simulink model "INPUT_autosar"  (R2019b)
settings: Solver=FixedStepAuto  StartTime=0.0  StopTime=10.0  RelTol=1e-3
undefined symbols (not defined in the file or in its folder): I_AN07_5V, I_AN08_5V, I_AN10_5V, I_SW01_L, I_SW02_L, I_SW03_L
libraries: ec5744lib x51, canmsglib x13
(part 1 of 2)
settings Model: Creator=12045  LastModifiedBy=12045
settings DataIOCC: ReturnWorkspaceOutputs=off
settings OptimizationCC: DefaultParameterBehavior=Inlined  EnhancedBackFolding=on  PassReuseOutputArgsAs=Individual arguments  ZeroExternalMemoryAtStartup=off  ZeroInternalMemoryAtStartup=off  OptimizeBlockOrder=speed  DifferentSizesBufferReuse=on  OptimizationCustomize=off  EfficientTunableParamExpr=on
settings DebuggingCC: ParameterTunabilityLossMsg=error  ArithmeticOperatorsInVariantConditions=warning
settings SFSimCC: MATLABDynamicMemAlloc=off  CustomCodeUndefinedFunction=UseInterfaceOnly
settings RTWCC: Description=AUTOSAR  SystemTargetFile=autosar.tlc  GenCodeOnly=on  TemplateMakefile=ert_default_tmf  GenerateReport=on  IncludeHyperlinkInReport=on  LaunchReport=on  GenerateTraceInfo=on  GenerateTraceReport=on  GenerateTraceReportSl=on  GenerateTraceReportSf=on  GenerateTraceReportEml=on
settings CodeAppCC: ForceParamTrailComments=on  IgnoreCustomStorageClasses=off  OperatorAnnotations=on  SimulinkDataObjDesc=on  SFDataObjDesc=on  InsertBlockDesc=on
settings STFCustomTargetCC: TargetLangStandard=C99 (ISO)  MultiwordLength=256  ParMdlRefBuildCompliant=on  CompOptLevelCompliant=on  IncludeMdlTerminateFcn=off  CombineOutputUpdateFcns=on  SuppressErrorStatus=on  ERTCustomFileBanners=on  SupportNonFinite=off  SupportComplex=off  SupportContinuousTime=off  SupportNonInlinedSFcns=off  RemoveResetFunc=on  MATLABClassNameForMDSCustomization=Simulink.SoftwareTarget.ERTCustomization  AutosarCompliant=on  UseToolchainInfoCompliant=on  LookupTableObjectStructAxisOrder=2,1,3,4,...  LUTObjectStructOrderEvenSpacing=Size,Table,Breakpoints  SystemTargetFile=autosar.tlc
settings ERTTargetCC: TargetLangStandard=C99 (ISO)  ConcurrentExecutionCompliant=off  IncludeMdlTerminateFcn=off  SuppressErrorStatus=on  SupportNonFinite=off  SupportComplex=off  ModelStepFunctionPrototypeControlCompliant=off  CPPClassGenCompliant=off  AutosarCompliant=on  LookupTableObjectStructAxisOrder=2,1,3,4,...  LUTObjectStructOrderEvenSpacing=Size,Table,Breakpoints  InlinedParameterPlacement=NonHierarchical  ERTCustomFileTemplate=example_file_process.tlc

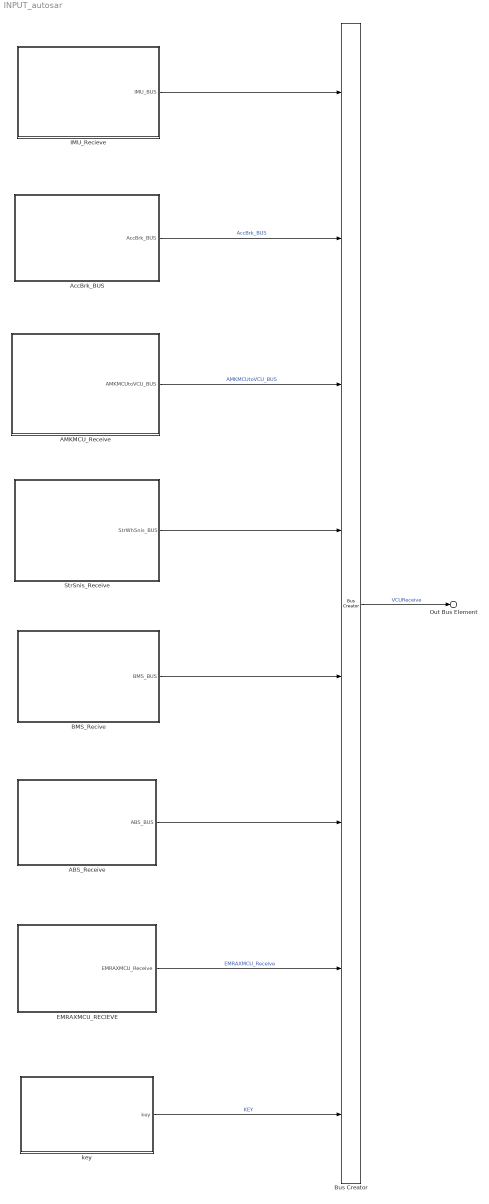
== system INPUT_autosar ==
  ABS_Receive : Subsystem  TreatAsAtomicUnit=on
  AMKMCU_Receive : Subsystem
  AccBrk_BUS : Subsystem
  BMS_Recive : Subsystem  TreatAsAtomicUnit=on
  Bus Creator : BusCreator  Inputs=8
  EMRAXMCU_RECIEVE : Subsystem  TreatAsAtomicUnit=on
  IMU_Recieve : Subsystem  TreatAsAtomicUnit=on
  StrSnis_Receive : Subsystem  TreatAsAtomicUnit=on
  key : Subsystem  TreatAsAtomicUnit=on
  Out Bus Element : Outport  PortName=INPUT_BUS  Element=INPUT_BUS
  wires:
  ABS_Receive/1(ABS_BUS) -> Bus Creator/6
  key/1(key) -> Bus Creator/8  "KEY"
  AMKMCU_Receive/1(AMKMCUtoVCU_BUS) -> Bus Creator/3  "AMKMCUtoVCU_BUS"
  BMS_Recive/1(BMS_BUS) -> Bus Creator/5
  AccBrk_BUS/1(AccBrk_BUS) -> Bus Creator/2  "AccBrk_BUS"
  IMU_Recieve/1(IMU_BUS) -> Bus Creator/1
  EMRAXMCU_RECIEVE/1(EMRAXMCU_Receive) -> Bus Creator/7  "EMRAXMCU_Receive"
  StrSnis_Receive/1(StrWhSnis_BUS) -> Bus Creator/4
  Bus Creator/1 -> Out Bus Element/1  "VCUReceive"

== system INPUT_autosar/ABS_Receive ==
  ABS_BUS_state : Subsystem  TreatAsAtomicUnit=on
  CANReceive3 : ec5744lib/RapidECU_U3/04CANCommunication/CANReceive  canmodule=0  canbuffer=16  canmessageid=1698  canmessagetype=Standard(11-bit ID)  datalength=8  sampletime=-1
      settings: SourceProductName=ECUCoder for MPC5744
  Terminator3 : Terminator
  ABS_BUS : Outport  VectorParamsAs1DForOutWhenUnconnected=off
  wires:
  CANReceive3/3 -> ABS_BUS_state/2(ID)
  CANReceive3/4 -> ABS_BUS_state/3(Msg)
  CANReceive3/1 -> ABS_BUS_state/Trigger
  ABS_BUS_state/1(ABS_BUS) -> ABS_BUS/1  "ABS_BUS"
  CANReceive3/5 -> Terminator3/1
  CANReceive3/2 -> ABS_BUS_state/1(CANOK)

== system INPUT_autosar/AMKMCU_Receive ==
  Bus Creator : BusCreator  Inputs=6
  FLAMKMCU : Subsystem
  FRAMKMCU : Subsystem
  AMKMCUtoVCU_BUS : Outport  VectorParamsAs1DForOutWhenUnconnected=off
  wires:
  Bus Creator/1 -> AMKMCUtoVCU_BUS/1
  FLAMKMCU/1(FLAMKMCUtoVCU1) -> Bus Creator/1
  FLAMKMCU/2(FLAMKMCUtoVCU2) -> Bus Creator/2  "FLAMKMCUtoVCU2"
  FLAMKMCU/3(FLAMKMCUtoVCU3) -> Bus Creator/3
  FRAMKMCU/1(FRAMKMCUtoVCU1) -> Bus Creator/4
  FRAMKMCU/2(FRAMKMCUtoVCU2) -> Bus Creator/5
  FRAMKMCU/3(FRAMKMCUtoVCU3) -> Bus Creator/6

== system INPUT_autosar/AccBrk_BUS ==
  Acc1 : ec5744lib/RapidECU_U3/01BasicInput/AnalogInput  channel=56:I_AN10_5V  sampletime=-1
      settings: SourceProductName=ECUCoder for MPC5744
  Acc2 : ec5744lib/RapidECU_U3/01BasicInput/AnalogInput  channel=53:I_AN07_5V  sampletime=-1
      settings: SourceProductName=ECUCoder for MPC5744
  Brk1 : ec5744lib/RapidECU_U3/01BasicInput/AnalogInput  channel=54:I_AN08_5V  sampletime=-1
      settings: SourceProductName=ECUCoder for MPC5744
  Bus Creator : BusCreator  Inputs=3
  AccBrk_BUS : Outport  VectorParamsAs1DForOutWhenUnconnected=off
  wires:
  Brk1/1 -> Bus Creator/2  "Brk1"
  Acc1/1 -> Bus Creator/1  "Acc1"
  Bus Creator/1 -> AccBrk_BUS/1
  Acc2/1 -> Bus Creator/3  "Acc2"

== system INPUT_autosar/BMS_Recive ==
  ABS_BUS_state : Subsystem  TreatAsAtomicUnit=on
  CANReceive3 : ec5744lib/RapidECU_U3/04CANCommunication/CANReceive  canmodule=0  canbuffer=16  canmessageid=1698  canmessagetype=Standard(11-bit ID)  datalength=8  sampletime=-1
      settings: SourceProductName=ECUCoder for MPC5744
  Terminator3 : Terminator
  BMS_BUS : Outport  VectorParamsAs1DForOutWhenUnconnected=off
  wires:
  ABS_BUS_state/1(BMS_BUS) -> BMS_BUS/1  "BMS_BUS"
  CANReceive3/3 -> ABS_BUS_state/2(ID)
  CANReceive3/1 -> ABS_BUS_state/Trigger
  CANReceive3/2 -> ABS_BUS_state/1(CANOK)
  CANReceive3/5 -> Terminator3/1
  CANReceive3/4 -> ABS_BUS_state/3(Msg)

== system INPUT_autosar/EMRAXMCU_RECIEVE ==
  Bus Creator2 : BusCreator  Inputs=2
  CANReceive1 : ec5744lib/RapidECU_U3/04CANCommunication/CANReceive  canmodule=0  canbuffer=1  canmessageid=218089455  canmessagetype=Extended(29-bit ID)  datalength=8  sampletime=-1
      settings: SourceProductName=ECUCoder for MPC5744
  CANReceive3 : ec5744lib/RapidECU_U3/04CANCommunication/CANReceive  canmodule=0  canbuffer=0  canmessageid=218089199  canmessagetype=Extended(29-bit ID)  datalength=8  sampletime=-1
      settings: SourceProductName=ECUCoder for MPC5744
  MCU_pwr : Subsystem  TreatAsAtomicUnit=on
  MCU_state : Subsystem  TreatAsAtomicUnit=on
  Terminator1 : Terminator
  Terminator3 : Terminator
  EMRAXMCU_Receive : Outport
  wires:
  CANReceive1/3 -> MCU_pwr/2(ID)
  CANReceive1/4 -> MCU_pwr/3(Msg)
  CANReceive1/2 -> MCU_pwr/1(CANOK)
  CANReceive3/1 -> MCU_state/Trigger
  CANReceive1/1 -> MCU_pwr/Trigger
  MCU_pwr/1(MCU_pwr) -> Bus Creator2/2  "MCU_pwr"
  CANReceive3/2 -> MCU_state/1(CANOK)
  CANReceive3/5 -> Terminator3/1
  CANReceive1/5 -> Terminator1/1
  MCU_state/1(Out1) -> Bus Creator2/1  "MCU_state"
  CANReceive3/3 -> MCU_state/2(ID)
  CANReceive3/4 -> MCU_state/3(Msg)
  Bus Creator2/1 -> EMRAXMCU_Receive/1

== system INPUT_autosar/IMU_Recieve ==
  CANReceive3 : ec5744lib/RapidECU_U3/04CANCommunication/CANReceive  canmodule=0  canbuffer=0  canmessageid=513  canmessagetype=Standard(11-bit ID)  datalength=8  sampletime=-1
      settings: SourceProductName=ECUCoder for MPC5744
  IMU_state : Subsystem  TreatAsAtomicUnit=on
  Terminator3 : Terminator
  IMU_BUS : Outport  VectorParamsAs1DForOutWhenUnconnected=off
  wires:
  CANReceive3/3 -> IMU_state/2(ID)
  CANReceive3/1 -> IMU_state/Trigger
  IMU_state/1(IMU_BUS) -> IMU_BUS/1  "IMU"
  CANReceive3/2 -> IMU_state/1(CANOK)
  CANReceive3/5 -> Terminator3/1
  CANReceive3/4 -> IMU_state/3(Msg)

== system INPUT_autosar/StrSnis_Receive ==
  CANReceive3 : ec5744lib/RapidECU_U3/04CANCommunication/CANReceive  canmodule=0  canbuffer=7  canmessageid=330  canmessagetype=Standard(11-bit ID)  datalength=8  sampletime=-1
      settings: SourceProductName=ECUCoder for MPC5744
  StrWhSnis_state : Subsystem  TreatAsAtomicUnit=on
  Terminator3 : Terminator
  StrWhSnis_BUS : Outport  VectorParamsAs1DForOutWhenUnconnected=off
  wires:
  CANReceive3/2 -> StrWhSnis_state/1(CANOK)
  CANReceive3/5 -> Terminator3/1
  StrWhSnis_state/1(IMU_BUS) -> StrWhSnis_BUS/1  "SWAS"
  CANReceive3/1 -> StrWhSnis_state/Trigger
  CANReceive3/4 -> StrWhSnis_state/3(Msg)
  CANReceive3/3 -> StrWhSnis_state/2(ID)

== system INPUT_autosar/key ==
  Bus Creator : BusCreator  Inputs=3
  Logical Operator : Logic  Operator=NOT  AllPortsSameDT=off  OutDataTypeStr=boolean
  MeaModule : ec5744lib/RapidECU_U3/07Calibration/MeaModule  signal=ignition
      settings: SourceProductName=ECUCoder for MPC5744
  SwitchInput : ec5744lib/RapidECU_U3/01BasicInput/SwitchInput  channel=6:I_SW01_L  sampletime=-1
      settings: SourceProductName=ECUCoder for MPC5744
  SwitchInput1 : ec5744lib/RapidECU_U3/01BasicInput/SwitchInput  channel=7:I_SW02_L  sampletime=-1
      settings: SourceProductName=ECUCoder for MPC5744
  SwitchInput2 : ec5744lib/RapidECU_U3/01BasicInput/SwitchInput  channel=8:I_SW03_L  sampletime=-1
      settings: SourceProductName=ECUCoder for MPC5744
  key : Outport  VectorParamsAs1DForOutWhenUnconnected=off
  wires:
  SwitchInput/1 -> Logical Operator/1  "Drive_ready"
  SwitchInput1/1 -> Bus Creator/1  "AMKCLDCON"
  Bus Creator/1 -> key/1
  MeaModule/1 -> Bus Creator/2  "ignition"
  Logical Operator/1 -> MeaModule/1
  SwitchInput2/1 -> Bus Creator/3  "HVCUTOFF"

== system INPUT_autosar/ABS_Receive/ABS_BUS_state ==
  CANOK : Inport
  ID : Inport  Port=2
  Msg : Inport  Port=3
  function : TriggerPort  TriggerType=function-call  VariantControl=(inherit)
  Bus Creator3 : BusCreator  Inputs=4
  IMU_state : Subsystem  TreatAsAtomicUnit=on
  ABS_BUS : Outport  VectorParamsAs1DForOutWhenUnconnected=off
  wires:
  IMU_state/3(ABS_WS_FL) -> Bus Creator3/3
  IMU_state/2(ABS_WS_RL) -> Bus Creator3/2
  IMU_state/1(ABS_WS_FR) -> Bus Creator3/1
  Bus Creator3/1 -> ABS_BUS/1
  ID/1 -> IMU_state/1(ID)
  CANOK/1 -> IMU_state/Enable
  Msg/1 -> IMU_state/2(Msg)
  IMU_state/4(ABS_WS_RR) -> Bus Creator3/4

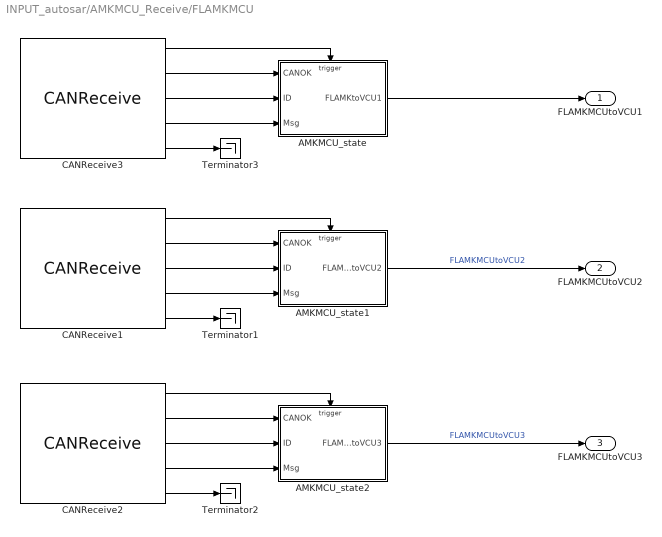
== system INPUT_autosar/AMKMCU_Receive/FLAMKMCU ==
  AMKMCU_state : Subsystem  TreatAsAtomicUnit=on
  AMKMCU_state1 : Subsystem  TreatAsAtomicUnit=on
  AMKMCU_state2 : Subsystem  TreatAsAtomicUnit=on
  CANReceive1 : ec5744lib/RapidECU_U3/04CANCommunication/CANReceive  canmodule=1  canbuffer=2  canmessageid=642  canmessagetype=Standard(11-bit ID)  datalength=8  sampletime=-1
      settings: SourceProductName=ECUCoder for MPC5744
  CANReceive2 : ec5744lib/RapidECU_U3/04CANCommunication/CANReceive  canmodule=1  canbuffer=3  canmessageid=644  canmessagetype=Standard(11-bit ID)  datalength=8  sampletime=-1
      settings: SourceProductName=ECUCoder for MPC5744
  CANReceive3 : ec5744lib/RapidECU_U3/04CANCommunication/CANReceive  canmodule=1  canbuffer=1  canmessageid=640  canmessagetype=Standard(11-bit ID)  datalength=8  sampletime=-1
      settings: SourceProductName=ECUCoder for MPC5744
  Terminator1 : Terminator
  Terminator2 : Terminator
  Terminator3 : Terminator
  FLAMKMCUtoVCU1 : Outport  VectorParamsAs1DForOutWhenUnconnected=off
  FLAMKMCUtoVCU2 : Outport  Port=2  VectorParamsAs1DForOutWhenUnconnected=off
  FLAMKMCUtoVCU3 : Outport  Port=3  VectorParamsAs1DForOutWhenUnconnected=off
  wires:
  CANReceive2/2 -> AMKMCU_state2/1(CANOK)
  CANReceive1/4 -> AMKMCU_state1/3(Msg)
  CANReceive3/5 -> Terminator3/1
  CANReceive1/3 -> AMKMCU_state1/2(ID)
  CANReceive1/1 -> AMKMCU_state1/Trigger
  CANReceive2/4 -> AMKMCU_state2/3(Msg)
  CANReceive3/3 -> AMKMCU_state/2(ID)
  CANReceive3/2 -> AMKMCU_state/1(CANOK)
  CANReceive2/3 -> AMKMCU_state2/2(ID)
  CANReceive1/2 -> AMKMCU_state1/1(CANOK)
  CANReceive1/5 -> Terminator1/1
  CANReceive3/4 -> AMKMCU_state/3(Msg)
  CANReceive2/5 -> Terminator2/1
  CANReceive3/1 -> AMKMCU_state/Trigger
  CANReceive2/1 -> AMKMCU_state2/Trigger
  AMKMCU_state2/1(FLAMKMCUtoVCU3) -> FLAMKMCUtoVCU3/1  "FLAMKMCUtoVCU3"
  AMKMCU_state/1(FLAMKtoVCU1) -> FLAMKMCUtoVCU1/1
  AMKMCU_state1/1(FLAMKMCUtoVCU2) -> FLAMKMCUtoVCU2/1  "FLAMKMCUtoVCU2"

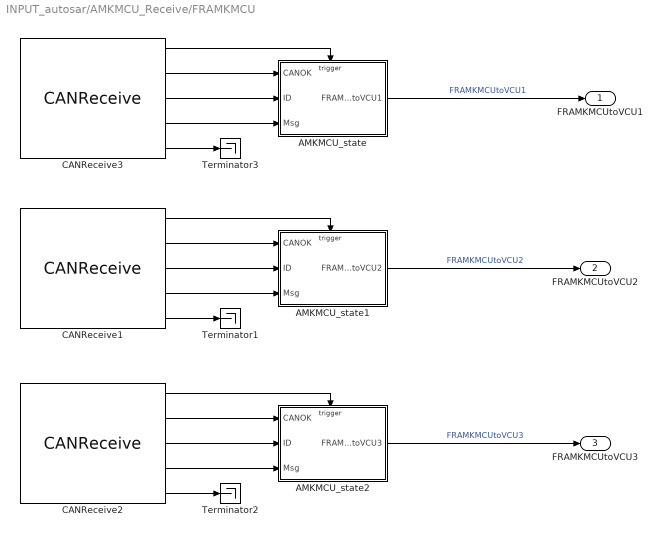
== system INPUT_autosar/AMKMCU_Receive/FRAMKMCU ==
  AMKMCU_state : Subsystem  TreatAsAtomicUnit=on
  AMKMCU_state1 : Subsystem  TreatAsAtomicUnit=on
  AMKMCU_state2 : Subsystem  TreatAsAtomicUnit=on
  CANReceive1 : ec5744lib/RapidECU_U3/04CANCommunication/CANReceive  canmodule=1  canbuffer=5  canmessageid=643  canmessagetype=Standard(11-bit ID)  datalength=8  sampletime=-1
      settings: SourceProductName=ECUCoder for MPC5744
  CANReceive2 : ec5744lib/RapidECU_U3/04CANCommunication/CANReceive  canmodule=1  canbuffer=6  canmessageid=387  canmessagetype=Standard(11-bit ID)  datalength=8  sampletime=-1
      settings: SourceProductName=ECUCoder for MPC5744
  CANReceive3 : ec5744lib/RapidECU_U3/04CANCommunication/CANReceive  canmodule=1  canbuffer=4  canmessageid=641  canmessagetype=Standard(11-bit ID)  datalength=8  sampletime=-1
      settings: SourceProductName=ECUCoder for MPC5744
  Terminator1 : Terminator
  Terminator2 : Terminator
  Terminator3 : Terminator
  FRAMKMCUtoVCU1 : Outport  VectorParamsAs1DForOutWhenUnconnected=off
  FRAMKMCUtoVCU2 : Outport  Port=2  VectorParamsAs1DForOutWhenUnconnected=off
  FRAMKMCUtoVCU3 : Outport  Port=3  VectorParamsAs1DForOutWhenUnconnected=off
  wires:
  AMKMCU_state1/1(FRAMKMCUtoVCU2) -> FRAMKMCUtoVCU2/1  "FRAMKMCUtoVCU2"
  AMKMCU_state/1(FRAMKMCUtoVCU1) -> FRAMKMCUtoVCU1/1  "FRAMKMCUtoVCU1"
  AMKMCU_state2/1(FRAMKMCUtoVCU3) -> FRAMKMCUtoVCU3/1  "FRAMKMCUtoVCU3"
  CANReceive2/1 -> AMKMCU_state2/Trigger
  CANReceive3/1 -> AMKMCU_state/Trigger
  CANReceive2/5 -> Terminator2/1
  CANReceive3/4 -> AMKMCU_state/3(Msg)
  CANReceive1/5 -> Terminator1/1
  CANReceive1/2 -> AMKMCU_state1/1(CANOK)
  CANReceive2/3 -> AMKMCU_state2/2(ID)
  CANReceive3/2 -> AMKMCU_state/1(CANOK)
  CANReceive3/3 -> AMKMCU_state/2(ID)
  CANReceive2/4 -> AMKMCU_state2/3(Msg)
  CANReceive1/1 -> AMKMCU_state1/Trigger
  CANReceive1/3 -> AMKMCU_state1/2(ID)
  CANReceive3/5 -> Terminator3/1
  CANReceive1/4 -> AMKMCU_state1/3(Msg)
  CANReceive2/2 -> AMKMCU_state2/1(CANOK)

== system INPUT_autosar/BMS_Recive/ABS_BUS_state ==
  CANOK : Inport
  ID : Inport  Port=2
  Msg : Inport  Port=3
  function : TriggerPort  TriggerType=function-call  VariantControl=(inherit)
  Bus Creator : BusCreator  Inputs=9
  IMU_state : Subsystem  TreatAsAtomicUnit=on
  BMS_BUS : Outport  VectorParamsAs1DForOutWhenUnconnected=off
  wires:
  Bus Creator/1 -> BMS_BUS/1
  ID/1 -> IMU_state/1(ID)
  CANOK/1 -> IMU_state/Enable
  Msg/1 -> IMU_state/2(Msg)
  IMU_state/1(BatAlmlv) -> Bus Creator/1
  IMU_state/2(BatLife) -> Bus Creator/2
  IMU_state/3(BatState) -> Bus Creator/3
  IMU_state/4(LSBAz) -> Bus Creator/4
  IMU_state/5(LSBVz) -> Bus Creator/5
  IMU_state/6(MSBAz) -> Bus Creator/6
  IMU_state/7(MSBVz) -> Bus Creator/7
  IMU_state/8(SOCz) -> Bus Creator/8
  IMU_state/9(SOHz) -> Bus Creator/9

== system INPUT_autosar/EMRAXMCU_RECIEVE/MCU_pwr ==
  CANOK : Inport
  ID : Inport  Port=2
  Msg : Inport  Port=3
  function : TriggerPort  TriggerType=function-call  VariantControl=(inherit)
  Bus Creator3 : BusCreator  Inputs=5
  MCU_VCUMeter1 : Subsystem  TreatAsAtomicUnit=on
  MCU_pwr : Outport
  wires:
  Bus Creator3/1 -> MCU_pwr/1
  Msg/1 -> MCU_VCUMeter1/2(Msg)
  CANOK/1 -> MCU_VCUMeter1/Enable
  ID/1 -> MCU_VCUMeter1/1(ID)
  MCU_VCUMeter1/1("AC_current ") -> Bus Creator3/1  "AC_current"
  MCU_VCUMeter1/2(MCU_temp) -> Bus Creator3/2  "MCU_temp"
  MCU_VCUMeter1/3(current) -> Bus Creator3/3  "current"
  MCU_VCUMeter1/4(motor_temp) -> Bus Creator3/4  "motor_temp"
  MCU_VCUMeter1/5(voltage) -> Bus Creator3/5  "voltage"

== system INPUT_autosar/EMRAXMCU_RECIEVE/MCU_state ==
  CANOK : Inport
  ID : Inport  Port=2
  Msg : Inport  Port=3
  function : TriggerPort  TriggerType=function-call  VariantControl=(inherit)
  Bus Creator3 : BusCreator  Inputs=15
  MCU_state : Subsystem  TreatAsAtomicUnit=on
  Out1 : Outport  VectorParamsAs1DForOutWhenUnconnected=off
  wires:
  Msg/1 -> MCU_state/2(Msg)
  CANOK/1 -> MCU_state/Enable
  ID/1 -> MCU_state/1(ID)
  Bus Creator3/1 -> Out1/1
  MCU_state/1(12V_error) -> Bus Creator3/1
  MCU_state/2(alarm) -> Bus Creator3/2
  MCU_state/3(undervol) -> Bus Creator3/3
  MCU_state/4(controller_ready) -> Bus Creator3/4
  MCU_state/5(MCU_temp_warn) -> Bus Creator3/5
  MCU_state/6(mode_cmd8) -> Bus Creator3/6
  MCU_state/7(motor_temp_warn) -> Bus Creator3/7
  MCU_state/8(overcur) -> Bus Creator3/8
  MCU_state/9(pow_lim_warn) -> Bus Creator3/9
  MCU_state/10(overvol) -> Bus Creator3/10
  MCU_state/11(precharge) -> Bus Creator3/11
  MCU_state/12(rotation_warn) -> Bus Creator3/12
  MCU_state/13(selfcech) -> Bus Creator3/13
  MCU_state/14(RPM) -> Bus Creator3/14
  MCU_state/15(torque) -> Bus Creator3/15

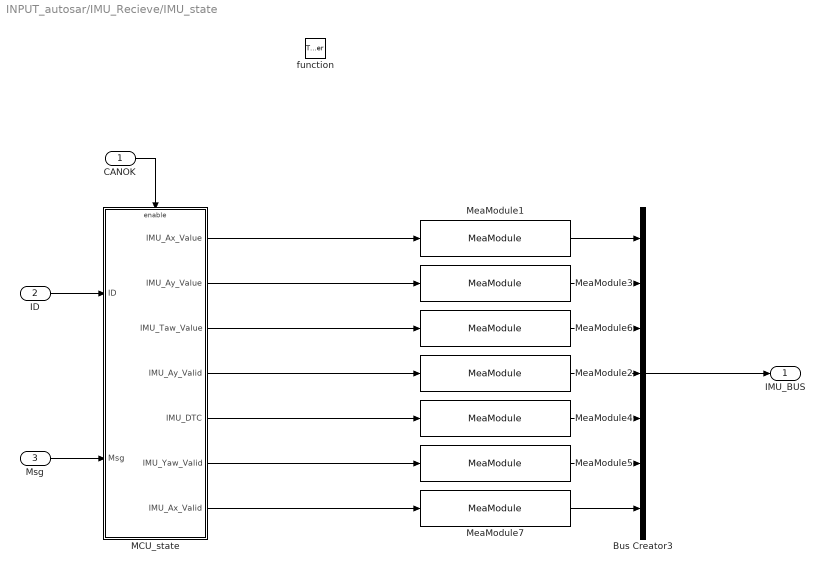
== system INPUT_autosar/IMU_Recieve/IMU_state ==
  CANOK : Inport
  ID : Inport  Port=2
  Msg : Inport  Port=3
  function : TriggerPort  TriggerType=function-call  VariantControl=(inherit)
  Bus Creator3 : BusCreator  Inputs=7
  MCU_state : Subsystem  TreatAsAtomicUnit=on
  MeaModule1 : ec5744lib/RapidECU_U3/07Calibration/MeaModule  signal=IMU_Ax_Value
      settings: SourceProductName=ECUCoder for MPC5744
  MeaModule2 : ec5744lib/RapidECU_U3/07Calibration/MeaModule  signal=IMU_Ay_Valid
      settings: SourceProductName=ECUCoder for MPC5744
  MeaModule3 : ec5744lib/RapidECU_U3/07Calibration/MeaModule  signal=IMU_Ay_Value
      settings: SourceProductName=ECUCoder for MPC5744
  MeaModule4 : ec5744lib/RapidECU_U3/07Calibration/MeaModule  signal=IMU_DTC
      settings: SourceProductName=ECUCoder for MPC5744
  MeaModule5 : ec5744lib/RapidECU_U3/07Calibration/MeaModule  signal=IMU_Yaw_Valid
      settings: SourceProductName=ECUCoder for MPC5744
  MeaModule6 : ec5744lib/RapidECU_U3/07Calibration/MeaModule  signal=IMU_Yaw_Value
      settings: SourceProductName=ECUCoder for MPC5744
  MeaModule7 : ec5744lib/RapidECU_U3/07Calibration/MeaModule  signal=IMU_Ax_Valid
      settings: SourceProductName=ECUCoder for MPC5744
  IMU_BUS : Outport  VectorParamsAs1DForOutWhenUnconnected=off
  wires:
  Msg/1 -> MCU_state/2(Msg)
  CANOK/1 -> MCU_state/Enable
  ID/1 -> MCU_state/1(ID)
  Bus Creator3/1 -> IMU_BUS/1
  MeaModule1/1 -> Bus Creator3/1
  MeaModule3/1 -> Bus Creator3/2
  MeaModule6/1 -> Bus Creator3/3
  MeaModule2/1 -> Bus Creator3/4
  MeaModule4/1 -> Bus Creator3/5
  MeaModule5/1 -> Bus Creator3/6
  MeaModule7/1 -> Bus Creator3/7
  MCU_state/1(IMU_Ax_Value) -> MeaModule1/1
  MCU_state/2(IMU_Ay_Value) -> MeaModule3/1
  MCU_state/3(IMU_Taw_Value) -> MeaModule6/1
  MCU_state/4(IMU_Ay_Valid) -> MeaModule2/1
  MCU_state/5(IMU_DTC) -> MeaModule4/1
  MCU_state/6(IMU_Yaw_Valid) -> MeaModule5/1
  MCU_state/7(IMU_Ax_Valid) -> MeaModule7/1

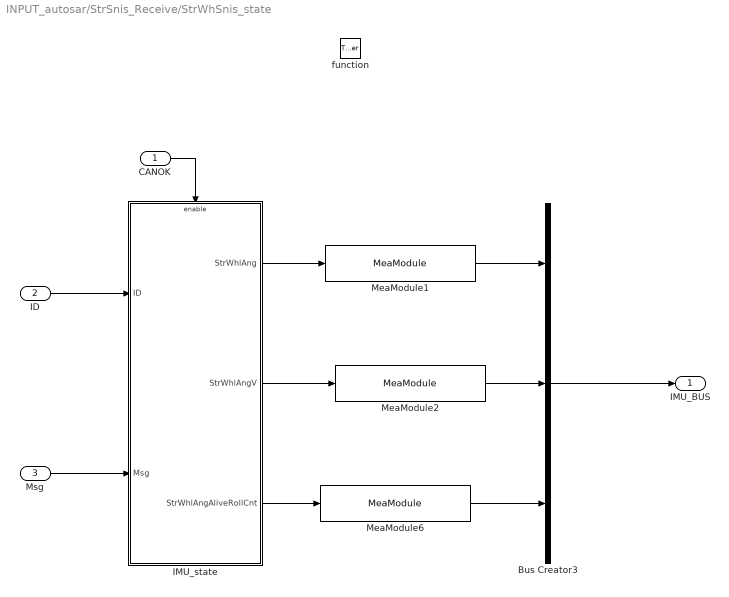
== system INPUT_autosar/StrSnis_Receive/StrWhSnis_state ==
  CANOK : Inport
  ID : Inport  Port=2
  Msg : Inport  Port=3
  function : TriggerPort  TriggerType=function-call  VariantControl=(inherit)
  Bus Creator3 : BusCreator  Inputs=3
  IMU_state : Subsystem  TreatAsAtomicUnit=on
  MeaModule1 : ec5744lib/RapidECU_U3/07Calibration/MeaModule  signal=StrWhlAng
      settings: SourceProductName=ECUCoder for MPC5744
  MeaModule2 : ec5744lib/RapidECU_U3/07Calibration/MeaModule  signal=StrWhlAngV
      settings: SourceProductName=ECUCoder for MPC5744
  MeaModule6 : ec5744lib/RapidECU_U3/07Calibration/MeaModule  signal=StrWhlAngAliveRollCnt
      settings: SourceProductName=ECUCoder for MPC5744
  IMU_BUS : Outport  VectorParamsAs1DForOutWhenUnconnected=off
  wires:
  Msg/1 -> IMU_state/2(Msg)
  CANOK/1 -> IMU_state/Enable
  ID/1 -> IMU_state/1(ID)
  IMU_state/1(StrWhlAng) -> MeaModule1/1
  Bus Creator3/1 -> IMU_BUS/1
  MeaModule1/1 -> Bus Creator3/1
  IMU_state/2(StrWhlAngV) -> MeaModule2/1
  IMU_state/3(StrWhlAngAliveRollCnt) -> MeaModule6/1
  MeaModule2/1 -> Bus Creator3/2
  MeaModule6/1 -> Bus Creator3/3

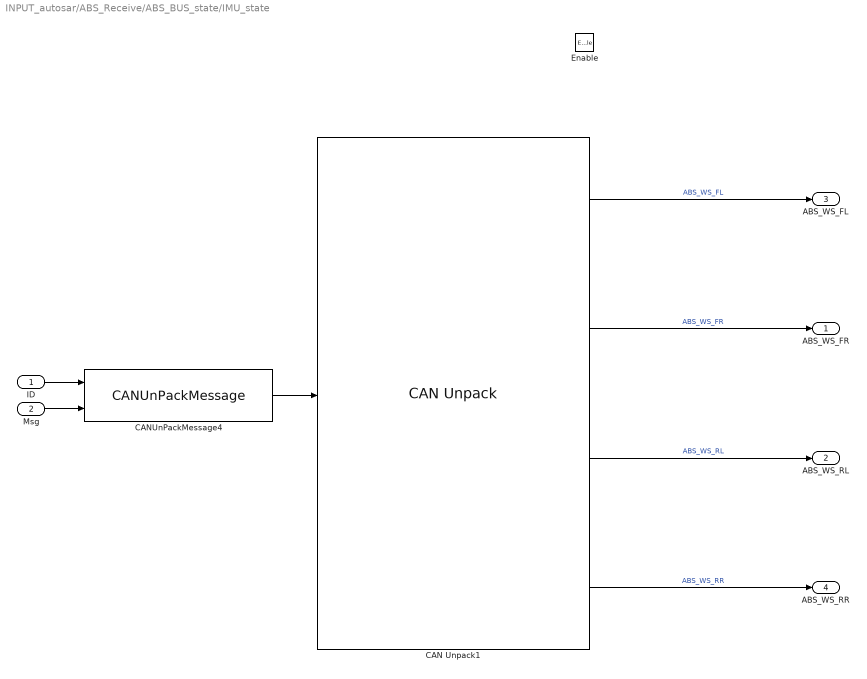
== system INPUT_autosar/ABS_Receive/ABS_BUS_state/IMU_state ==
  ID : Inport
  Msg : Inport  Port=2
  Enable : EnablePort
  CAN Unpack1 : canmsglib/CAN Unpack  CANdbFile=d:\Users\YJR\Desktop\DBC\Abs_Dev_Dbc_20240603_NingYuan.dbc  MsgList=(none)  MsgName=ABS_Basic_Msg2  MsgIDType=Standard (11-bit identifier)  MsgIdentifier=1698  MsgLength=8  SignalInfo={'WS_FL','8','16','BE','signed','Standard','0','1.406250e-02','0','-4.608000e+02','4.607859e+02';'WS_FR','24','16','BE','signed','Standard','0','1.406250e-02','0','-4.608000e+02','4.607859e+02';'WS_RL','40','16','BE','signed','Standard','0','1.406250e-02','0','-4.608000e+02','4.607859e+02';'WS_RR','56','16','BE','signed','Standard','0','1.406250e-02','0','-4.608000e+02','4.607859e+02'}  IDPort=off  TimestampPort=off  ErrorPort=off  RemotePort=off  LengthPort=off  StatusPort=off  ApplyMinMax=off
      settings: SourceProductName=Simulink Real-Time  SourceProductBaseCode=XP  DataFormat=CANdb specified signals
  CANUnPackMessage4 : ec5744lib/RapidECU_U3/04CANCommunication/CANUnPackMessage  datalength=8  canmessagetype=Standard(11-bit ID)  sampletime=-1
      settings: SourceProductName=ECUCoder for MPC5744
  ABS_WS_FR : Outport  VectorParamsAs1DForOutWhenUnconnected=off
  ABS_WS_RL : Outport  Port=2  VectorParamsAs1DForOutWhenUnconnected=off
  ABS_WS_FL : Outport  Port=3  VectorParamsAs1DForOutWhenUnconnected=off
  ABS_WS_RR : Outport  Port=4  VectorParamsAs1DForOutWhenUnconnected=off
  wires:
  CAN Unpack1/3 -> ABS_WS_RL/1  "ABS_WS_RL"
  CAN Unpack1/2 -> ABS_WS_FR/1  "ABS_WS_FR"
  CAN Unpack1/1 -> ABS_WS_FL/1  "ABS_WS_FL"
  CANUnPackMessage4/1 -> CAN Unpack1/1
  ID/1 -> CANUnPackMessage4/1
  Msg/1 -> CANUnPackMessage4/2
  CAN Unpack1/4 -> ABS_WS_RR/1  "ABS_WS_RR"

== system INPUT_autosar/AMKMCU_Receive/FLAMKMCU/AMKMCU_state ==
  CANOK : Inport
  ID : Inport  Port=2
  Msg : Inport  Port=3
  function : TriggerPort  TriggerType=function-call  VariantControl=(inherit)
  MCU_state : Subsystem  TreatAsAtomicUnit=on
  FLAMKtoVCU1 : Outport  VectorParamsAs1DForOutWhenUnconnected=off
  wires:
  Msg/1 -> MCU_state/2(Msg)
  CANOK/1 -> MCU_state/Enable
  ID/1 -> MCU_state/1(ID)
  MCU_state/1(FLAMKMCUtoVCU1) -> FLAMKtoVCU1/1

== system INPUT_autosar/AMKMCU_Receive/FLAMKMCU/AMKMCU_state1 ==
  CANOK : Inport
  ID : Inport  Port=2
  Msg : Inport  Port=3
  function : TriggerPort  TriggerType=function-call  VariantControl=(inherit)
  Bus Creator : BusCreator  Inputs=2
  MCU_state : Subsystem  TreatAsAtomicUnit=on
  FLAMKMCUtoVCU2 : Outport  VectorParamsAs1DForOutWhenUnconnected=off
  wires:
  MCU_state/2(MCFL_ErrorInfo) -> Bus Creator/2
  MCU_state/1(MCFL_DiagnosticNum) -> Bus Creator/1
  Bus Creator/1 -> FLAMKMCUtoVCU2/1
  ID/1 -> MCU_state/1(ID)
  CANOK/1 -> MCU_state/Enable
  Msg/1 -> MCU_state/2(Msg)

== system INPUT_autosar/AMKMCU_Receive/FLAMKMCU/AMKMCU_state2 ==
  CANOK : Inport
  ID : Inport  Port=2
  Msg : Inport  Port=3
  function : TriggerPort  TriggerType=function-call  VariantControl=(inherit)
  Bus Creator : BusCreator  Inputs=3
  MCU_state : Subsystem  TreatAsAtomicUnit=on
  FLAMKMCUtoVCU3 : Outport  VectorParamsAs1DForOutWhenUnconnected=off
  wires:
  Msg/1 -> MCU_state/2(Msg)
  CANOK/1 -> MCU_state/Enable
  ID/1 -> MCU_state/1(ID)
  Bus Creator/1 -> FLAMKMCUtoVCU3/1  "Bus Creator"
  MCU_state/1(MCFL_TempIGBT) -> Bus Creator/1
  MCU_state/2(MCFL_TempInverter) -> Bus Creator/2
  MCU_state/3(MCFL_TempMotor) -> Bus Creator/3

== system INPUT_autosar/AMKMCU_Receive/FRAMKMCU/AMKMCU_state ==
  CANOK : Inport
  ID : Inport  Port=2
  Msg : Inport  Port=3
  function : TriggerPort  TriggerType=function-call  VariantControl=(inherit)
  Bus Creator : BusCreator  Inputs=12
  MCU_state : Subsystem  TreatAsAtomicUnit=on
  FRAMKMCUtoVCU1 : Outport  VectorParamsAs1DForOutWhenUnconnected=off
  wires:
  ID/1 -> MCU_state/1(ID)
  CANOK/1 -> MCU_state/Enable
  Msg/1 -> MCU_state/2(Msg)
  MCU_state/1(MCFR_ActualTorque) -> Bus Creator/1
  MCU_state/2(MCFR_ActualVelocity) -> Bus Creator/2
  MCU_state/3(MCFR_DCVoltage) -> Bus Creator/3
  MCU_state/4(MCFR_bDCOn) -> Bus Creator/4
  MCU_state/5(MCFR_bDerating) -> Bus Creator/5
  MCU_state/6(MCFR_bError) -> Bus Creator/6
  MCU_state/7(MCFR_bInverterOn) -> Bus Creator/7
  MCU_state/8(MCFR_bQuitDCOn) -> Bus Creator/8
  MCU_state/9(MCFR_bQuitInverterOn) -> Bus Creator/9
  MCU_state/10(MCFR_bReserve) -> Bus Creator/10
  MCU_state/11(MCFR_bSystemReady) -> Bus Creator/11
  MCU_state/12(MCFR_bWarn) -> Bus Creator/12
  Bus Creator/1 -> FRAMKMCUtoVCU1/1

== system INPUT_autosar/AMKMCU_Receive/FRAMKMCU/AMKMCU_state1 ==
  CANOK : Inport
  ID : Inport  Port=2
  Msg : Inport  Port=3
  function : TriggerPort  TriggerType=function-call  VariantControl=(inherit)
  Bus Creator : BusCreator  Inputs=2
  MCU_state : Subsystem  TreatAsAtomicUnit=on
  FRAMKMCUtoVCU2 : Outport  VectorParamsAs1DForOutWhenUnconnected=off
  wires:
  Msg/1 -> MCU_state/2(Msg)
  CANOK/1 -> MCU_state/Enable
  ID/1 -> MCU_state/1(ID)
  Bus Creator/1 -> FRAMKMCUtoVCU2/1
  MCU_state/1(MCFR_DiagnosticNum) -> Bus Creator/1
  MCU_state/2(MCFR_ErrorInfo) -> Bus Creator/2

== system INPUT_autosar/AMKMCU_Receive/FRAMKMCU/AMKMCU_state2 ==
  CANOK : Inport
  ID : Inport  Port=2
  Msg : Inport  Port=3
  function : TriggerPort  TriggerType=function-call  VariantControl=(inherit)
  Bus Creator : BusCreator  Inputs=3
  MCU_state : Subsystem  TreatAsAtomicUnit=on
  FRAMKMCUtoVCU3 : Outport  VectorParamsAs1DForOutWhenUnconnected=off
  wires:
  Bus Creator/1 -> FRAMKMCUtoVCU3/1
  ID/1 -> MCU_state/1(ID)
  CANOK/1 -> MCU_state/Enable
  Msg/1 -> MCU_state/2(Msg)
  MCU_state/1(MCFR_TempIGBT) -> Bus Creator/1
  MCU_state/2(MCFR_TempInverter) -> Bus Creator/2
  MCU_state/3(MCFR_TempMotor) -> Bus Creator/3

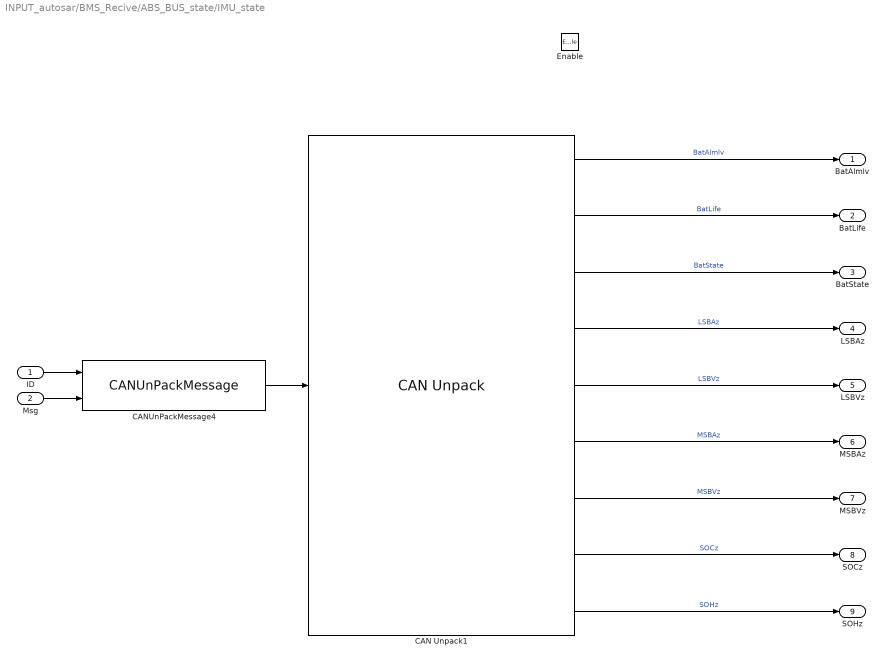
== system INPUT_autosar/BMS_Recive/ABS_BUS_state/IMU_state ==
  ID : Inport
  Msg : Inport  Port=2
  Enable : EnablePort
  CAN Unpack1 : canmsglib/CAN Unpack  CANdbFile=d:\Users\YJR\Desktop\DBC\bms.dbc  MsgList=(none)  MsgName=BMS_HCU_INFO  MsgIDType=Extended (29-bit identifier)  MsgIdentifier=408961267  MsgLength=8  SignalInfo={'BatAlmlv','52','4','LE','signed','Standard','0','1','0','0','4';'BatLife','56','8','LE','signed','Standard','0','1','0','0','255';'BatState','48','4','LE','signed','Standard','0','1','0','0','7';'LSBAz','24','8','LE','signed','Standard','0','1.000000e-01','-1000','-1.012800e+03','-9.873000e+02';'LSBVz','8','8','LE','unsigned','Standard','0','1.000000e-01','0','0','9000';'MSBAz','16','8','LE','unsigned','Standard','0','1.000000e-01','-1000','-1000','-9.745000e+02';'MSBVz','0','8','LE','unsigned','Standard','0','1.000000e-01','0','0','9000';'SOCz','32','8','LE','signed','Standard','0','1','0','0','100';'SOHz','40','8','LE','signed','Standard','0','1','0','0','100'}  IDPort=off  TimestampPort=off  ErrorPort=off  RemotePort=off  LengthPort=off  StatusPort=off  ApplyMinMax=off
      settings: SourceProductName=Simulink Real-Time  SourceProductBaseCode=XP  DataFormat=CANdb specified signals
  CANUnPackMessage4 : ec5744lib/RapidECU_U3/04CANCommunication/CANUnPackMessage  datalength=8  canmessagetype=Standard(11-bit ID)  sampletime=-1
      settings: SourceProductName=ECUCoder for MPC5744
  BatAlmlv : Outport  VectorParamsAs1DForOutWhenUnconnected=off
  BatLife : Outport  Port=2  VectorParamsAs1DForOutWhenUnconnected=off
  BatState : Outport  Port=3  VectorParamsAs1DForOutWhenUnconnected=off
  LSBAz : Outport  Port=4  VectorParamsAs1DForOutWhenUnconnected=off
  LSBVz : Outport  Port=5  VectorParamsAs1DForOutWhenUnconnected=off
  MSBAz : Outport  Port=6  VectorParamsAs1DForOutWhenUnconnected=off
  MSBVz : Outport  Port=7  VectorParamsAs1DForOutWhenUnconnected=off
  SOCz : Outport  Port=8  VectorParamsAs1DForOutWhenUnconnected=off
  SOHz : Outport  Port=9  VectorParamsAs1DForOutWhenUnconnected=off
  wires:
  CANUnPackMessage4/1 -> CAN Unpack1/1
  ID/1 -> CANUnPackMessage4/1
  Msg/1 -> CANUnPackMessage4/2
  CAN Unpack1/1 -> BatAlmlv/1  "BatAlmlv"
  CAN Unpack1/2 -> BatLife/1  "BatLife"
  CAN Unpack1/3 -> BatState/1  "BatState"
  CAN Unpack1/4 -> LSBAz/1  "LSBAz"
  CAN Unpack1/5 -> LSBVz/1  "LSBVz"
  CAN Unpack1/6 -> MSBAz/1  "MSBAz"
  CAN Unpack1/7 -> MSBVz/1  "MSBVz"
  CAN Unpack1/8 -> SOCz/1  "SOCz"
  CAN Unpack1/9 -> SOHz/1  "SOHz"

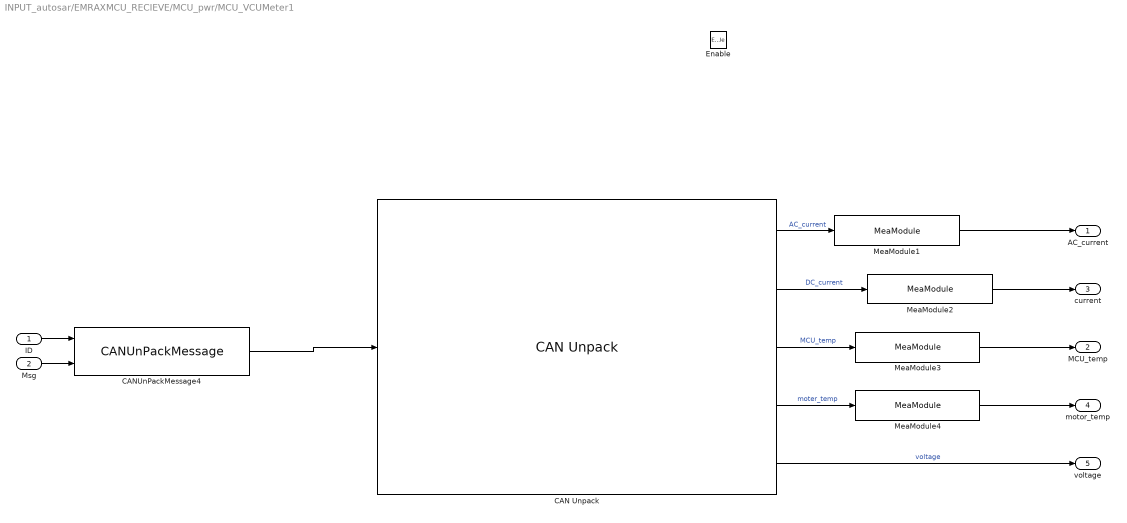
== system INPUT_autosar/EMRAXMCU_RECIEVE/MCU_pwr/MCU_VCUMeter1 ==
  ID : Inport
  Msg : Inport  Port=2
  Enable : EnablePort
  CAN Unpack : canmsglib/CAN Unpack  CANdbFile=E:\candbc\MCU_No1.dbc  MsgList=(none)  MsgName=MCU2VCU2_ID1  MsgIDType=Extended (29-bit identifier)  MsgIdentifier=218089455  MsgLength=8  SignalInfo={'MCU2VCU2_Current_AC_Feedback_ID1','48','16','LE','unsigned','Standard','0','1.000000e-01','-1600','-1600','1600';'MCU2VCU2_Current_DC_feedback_ID1','32','16','LE','unsigned','Standard','0','1.000000e-01','-1600','-1600','1600';'MCU2VCU2_MCU_Temp_ID1','0','8','LE','unsigned','Standard','0','1','-50','-50','200';'MCU2VCU2_Motor_Temp_ID1','8','8','LE','unsigned','Standard','0','1','-50','-50','200';'MCU2VCU2_Voltage_Feedback_ID1','16','16','LE','unsigned','Standard','0','1.000000e-01','0','0','1000'}  IDPort=off  TimestampPort=off  ErrorPort=off  RemotePort=off  LengthPort=off  StatusPort=off  ApplyMinMax=off
      settings: SourceProductName=Vehicle Network Toolbox  SourceProductBaseCode=VN  DataFormat=CANdb specified signals
  CANUnPackMessage4 : ec5744lib/RapidECU_U3/04CANCommunication/CANUnPackMessage  datalength=8  canmessagetype=Extended(29-bit ID)  sampletime=-1
      settings: SourceProductName=ECUCoder for MPC5744
  MeaModule1 : ec5744lib/RapidECU_U3/07Calibration/MeaModule  signal=AC_current
      settings: SourceProductName=ECUCoder for MPC5744
  MeaModule2 : ec5744lib/RapidECU_U3/07Calibration/MeaModule  signal=DC_current
      settings: SourceProductName=ECUCoder for MPC5744
  MeaModule3 : ec5744lib/RapidECU_U3/07Calibration/MeaModule  signal=MCU_Temp
      settings: SourceProductName=ECUCoder for MPC5744
  MeaModule4 : ec5744lib/RapidECU_U3/07Calibration/MeaModule  signal=motor_Temp
      settings: SourceProductName=ECUCoder for MPC5744
  "AC_current " : Outport
  MCU_temp : Outport  Port=2
  current : Outport  Port=3
  motor_temp : Outport  Port=4
  voltage : Outport  Port=5
  wires:
  Msg/1 -> CANUnPackMessage4/2
  ID/1 -> CANUnPackMessage4/1
  CANUnPackMessage4/1 -> CAN Unpack/1
  CAN Unpack/1 -> MeaModule1/1  "AC_current"
  CAN Unpack/5 -> voltage/1  "voltage"
  CAN Unpack/4 -> MeaModule4/1  "moter_temp"
  MeaModule1/1 -> "AC_current "/1
  MeaModule2/1 -> current/1
  CAN Unpack/3 -> MeaModule3/1  "MCU_temp"
  CAN Unpack/2 -> MeaModule2/1  "DC_current"
  MeaModule3/1 -> MCU_temp/1
  MeaModule4/1 -> motor_temp/1

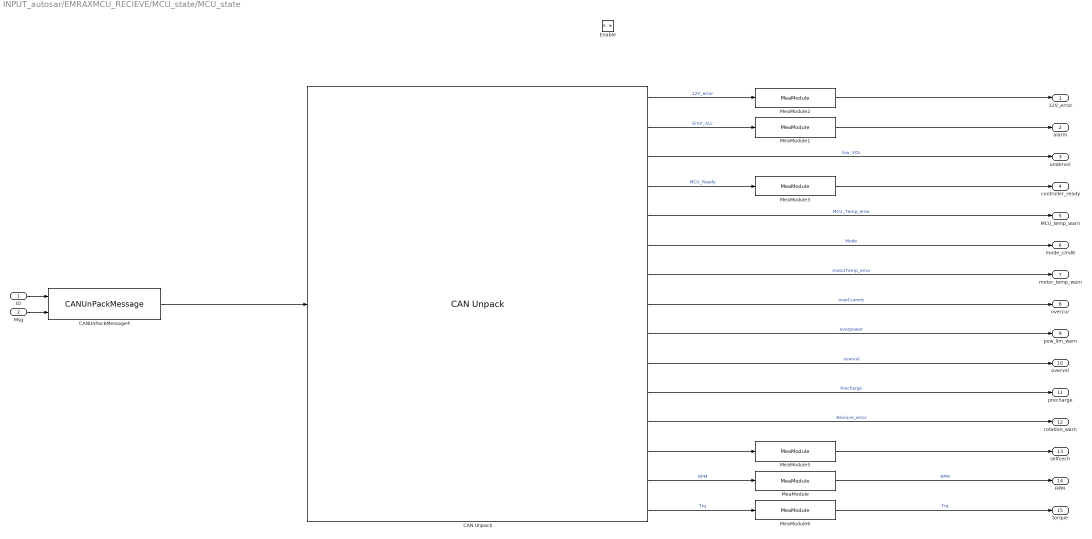
== system INPUT_autosar/EMRAXMCU_RECIEVE/MCU_state/MCU_state ==
  ID : Inport
  Msg : Inport  Port=2
  Enable : EnablePort
  CAN Unpack : canmsglib/CAN Unpack  CANdbFile=E:\candbc\MCU_No1.dbc  MsgList=(none)  MsgName=MCU2VCU1_ID1  MsgIDType=Extended (29-bit identifier)  MsgIdentifier=218089199  MsgLength=8  SignalInfo={'MCU2VCU1_12V_error_ID1','45','1','LE','unsigned','Standard','0','1','0','0','1';'MCU2VCU1_Error_All_ID1','56','2','LE','unsigned','Standard','0','1','0','0','3';'MCU2VCU1_LowVoltage_error_ID1','46','1','LE','unsigned','Standard','0','1','0','0','1';'MCU2VCU1_MCU_Ready_ID1','40','1','LE','unsigned','Standard','0','1','0','0','1';'MCU2VCU1_MCU_Temp_error_ID1','48','1','LE','unsigned','Standard','0','1','0','0','1';'MCU2VCU1_Mode_Feedback_ID1','32','8','LE','unsigned','Standard','0','1','0','0','255';'MCU2VCU1_MotorTemp_error_ID1','49','1','LE','unsigned','Standard','0','1','0','0','1';'MCU2VCU1_OverCurrent_error_ID1','43','1','LE','unsigned','Standard','0','1','0','0','1';'MCU2VCU1_OverPower_error_ID1','47','1','LE','unsigned','Standard','0','1','0','0','1';'MCU2VCU1_OverVoltage_error_ID1','44','1','LE','unsigned','Standard','0','1','0','0','1';'MCU2VCU1_PrechargeState_ID1','41','1','LE','unsigned','Standard','0','1','0','0','1';'MCU2VCU1_Reslove_Error_ID1','42','1','LE','unsigned','Standard','0','1','0','0','1';'MCU2VCU1_Selfcheck_ID1','55','1','LE','unsigned','Standard','0','1','0','0','1';'MCU2VCU1_Speed_Feedback_ID1','0','16','LE','unsigned','Standard','0','5.000000e-01','-10000','-10000','10000';'MCU2VCU1_Torque_Feedback_ID1','16','16','LE','unsigned','Standard','0','1','0','0','1000'}  IDPort=off  TimestampPort=off  ErrorPort=off  RemotePort=off  LengthPort=off  StatusPort=off  ApplyMinMax=off
      settings: SourceProductName=Vehicle Network Toolbox  SourceProductBaseCode=VN  DataFormat=CANdb specified signals
  CANUnPackMessage4 : ec5744lib/RapidECU_U3/04CANCommunication/CANUnPackMessage  datalength=8  canmessagetype=Extended(29-bit ID)  sampletime=-1
      settings: SourceProductName=ECUCoder for MPC5744
  MeaModule : ec5744lib/RapidECU_U3/07Calibration/MeaModule  signal=RPM
      settings: SourceProductName=ECUCoder for MPC5744
  MeaModule1 : ec5744lib/RapidECU_U3/07Calibration/MeaModule  signal=alarm
      settings: SourceProductName=ECUCoder for MPC5744
  MeaModule2 : ec5744lib/RapidECU_U3/07Calibration/MeaModule  signal=L12V_error
      settings: SourceProductName=ECUCoder for MPC5744
  MeaModule3 : ec5744lib/RapidECU_U3/07Calibration/MeaModule  signal=controller_ready
      settings: SourceProductName=ECUCoder for MPC5744
  MeaModule5 : ec5744lib/RapidECU_U3/07Calibration/MeaModule  signal=selfcheck
      settings: SourceProductName=ECUCoder for MPC5744
  MeaModule6 : ec5744lib/RapidECU_U3/07Calibration/MeaModule  signal=trq
      settings: SourceProductName=ECUCoder for MPC5744
  12V_error : Outport
  alarm : Outport  Port=2
  undervol : Outport  Port=3
  controller_ready : Outport  Port=4
  MCU_temp_warn : Outport  Port=5
  mode_cmd8 : Outport  Port=6
  motor_temp_warn : Outport  Port=7
  overcur : Outport  Port=8
  pow_lim_warn : Outport  Port=9
  overvol : Outport  Port=10
  precharge : Outport  Port=11
  rotation_warn : Outport  Port=12
  selfcech : Outport  Port=13
  RPM : Outport  Port=14
  torque : Outport  Port=15
  wires:
  Msg/1 -> CANUnPackMessage4/2
  ID/1 -> CANUnPackMessage4/1
  CANUnPackMessage4/1 -> CAN Unpack/1
  MeaModule/1 -> RPM/1  "RPM"
  MeaModule1/1 -> alarm/1
  MeaModule2/1 -> 12V_error/1
  MeaModule3/1 -> controller_ready/1
  MeaModule5/1 -> selfcech/1
  MeaModule6/1 -> torque/1  "Trq"
  CAN Unpack/14 -> MeaModule/1  "RPM"
  CAN Unpack/15 -> MeaModule6/1  "Trq"
  CAN Unpack/13 -> MeaModule5/1
  CAN Unpack/11 -> precharge/1  "Precharge"
  CAN Unpack/10 -> overvol/1  "overvol"
  CAN Unpack/9 -> pow_lim_warn/1  "overpower"
  CAN Unpack/8 -> overcur/1  "overCurrent"
  CAN Unpack/7 -> motor_temp_warn/1  "motorTemp_error"
  CAN Unpack/6 -> mode_cmd8/1  "Mode"
  CAN Unpack/5 -> MCU_temp_warn/1  "MCU_Temp_error"
  CAN Unpack/4 -> MeaModule3/1  "MCU_Ready"
  CAN Unpack/3 -> undervol/1  "low_VOL"
  CAN Unpack/2 -> MeaModule1/1  "Error_ALL"
  CAN Unpack/1 -> MeaModule2/1  "12V_error"
  CAN Unpack/12 -> rotation_warn/1  "Reslove_error"

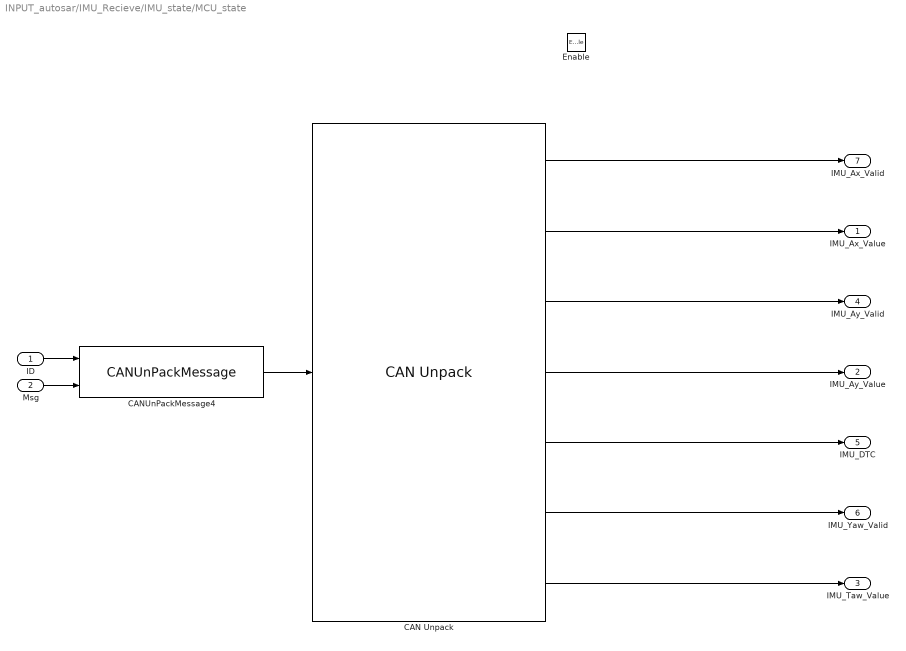
== system INPUT_autosar/IMU_Recieve/IMU_state/MCU_state ==
  ID : Inport
  Msg : Inport  Port=2
  Enable : EnablePort
  CAN Unpack : canmsglib/CAN Unpack  CANdbFile=d:\Users\YJR\Desktop\IMU.dbc  MsgList=(none)  MsgName=IMU  MsgIDType=Standard (11-bit identifier)  MsgIdentifier=513  MsgLength=8  SignalInfo={'IMU_Ax_Valid','1','1','LE','unsigned','Standard','0','1','0','-Inf','Inf';'IMU_Ax_Value','40','16','LE','unsigned','Standard','0','1.500000e-04','-4.915200e+00','-Inf','Inf';'IMU_Ay_Valid','2','1','LE','unsigned','Standard','0','1','0','-Inf','Inf';'IMU_Ay_Value','24','16','LE','unsigned','Standard','0','1.500000e-04','-4.915200e+00','-Inf','Inf';'IMU_DTC','4','4','LE','unsigned','Standard','0','1','0','-Inf','Inf';'IMU_Yaw_Valid','3','1','LE','unsigned','Standard','0','1','0','-Inf','Inf';'IMU_Yaw_Value','8','16','LE','unsigned','Standard','0','5.710000e-03','-1.872400e+02','-Inf','Inf'}  IDPort=off  TimestampPort=off  ErrorPort=off  RemotePort=off  LengthPort=off  StatusPort=off  ApplyMinMax=off
      settings: SourceProductName=Simulink Real-Time  SourceProductBaseCode=XP  DataFormat=CANdb specified signals
  CANUnPackMessage4 : ec5744lib/RapidECU_U3/04CANCommunication/CANUnPackMessage  datalength=8  canmessagetype=Standard(11-bit ID)  sampletime=-1
      settings: SourceProductName=ECUCoder for MPC5744
  IMU_Ax_Value : Outport  VectorParamsAs1DForOutWhenUnconnected=off
  IMU_Ay_Value : Outport  Port=2  VectorParamsAs1DForOutWhenUnconnected=off
  IMU_Taw_Value : Outport  Port=3  VectorParamsAs1DForOutWhenUnconnected=off
  IMU_Ay_Valid : Outport  Port=4  VectorParamsAs1DForOutWhenUnconnected=off
  IMU_DTC : Outport  Port=5  VectorParamsAs1DForOutWhenUnconnected=off
  IMU_Yaw_Valid : Outport  Port=6  VectorParamsAs1DForOutWhenUnconnected=off
  IMU_Ax_Valid : Outport  Port=7  VectorParamsAs1DForOutWhenUnconnected=off
  wires:
  Msg/1 -> CANUnPackMessage4/2
  ID/1 -> CANUnPackMessage4/1
  CANUnPackMessage4/1 -> CAN Unpack/1
  CAN Unpack/1 -> IMU_Ax_Valid/1
  CAN Unpack/2 -> IMU_Ax_Value/1
  CAN Unpack/3 -> IMU_Ay_Valid/1
  CAN Unpack/4 -> IMU_Ay_Value/1
  CAN Unpack/5 -> IMU_DTC/1
  CAN Unpack/7 -> IMU_Taw_Value/1
  CAN Unpack/6 -> IMU_Yaw_Valid/1

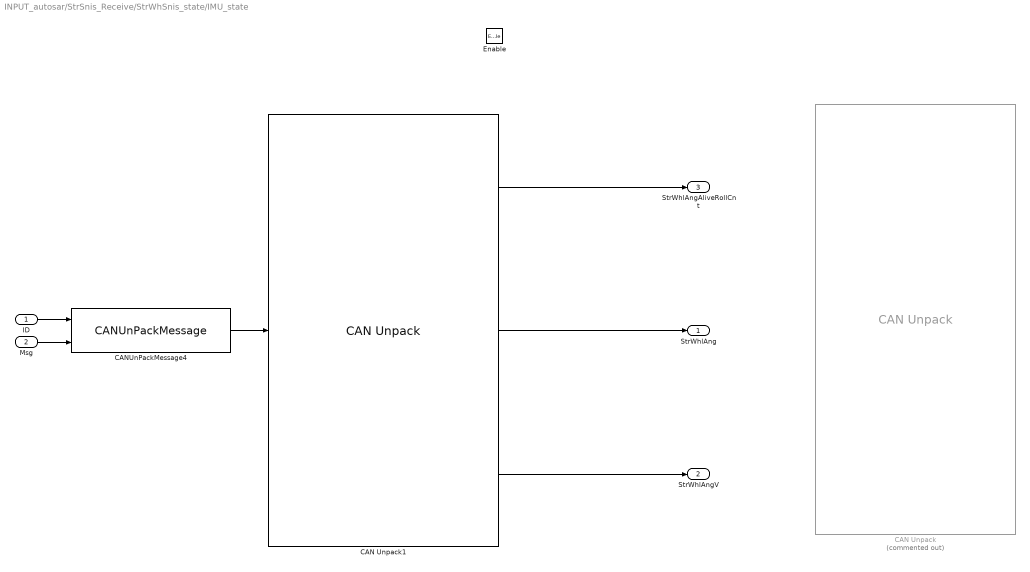
== system INPUT_autosar/StrSnis_Receive/StrWhSnis_state/IMU_state ==
  ID : Inport
  Msg : Inport  Port=2
  Enable : EnablePort
  CAN Unpack : canmsglib/CAN Unpack  Commented=on  CANdbFile=d:\Users\YJR\Desktop\DBC\SWAS_3.dbc  MsgList=(none)  MsgName=PPEI_Steering_Wheel_Angle  MsgIDType=Standard (11-bit identifier)  MsgIdentifier=330  MsgLength=8  SignalInfo={'SAS_CheckSum','36','4','LE','unsigned','Standard','0','1','0','-Inf','Inf';'SAS_MassageCounter','32','4','LE','unsigned','Standard','0','1','0','0','15';'SAS_TrimmingFlag','26','1','LE','unsigned','Standard','0','1','0','0','255';'StrWhAng','8','16','BE','unsigned','Standard','0','1','0','0','65535';'StrWhAngV','16','8','LE','unsigned','Standard','0','1','0','0','1';'StrWhlAngSenCalFlag','25','1','LE','unsigned','Standard','0','1','0','0','3';'StrngWhlAngSnsrFailFlag','24','1','LE','unsigned','Standard','0','1','0','0','1'}  IDPort=off  TimestampPort=off  ErrorPort=off  RemotePort=off  LengthPort=off  StatusPort=off  ApplyMinMax=off
      settings: SourceProductName=Simulink Real-Time  SourceProductBaseCode=XP  DataFormat=CANdb specified signals
  CAN Unpack1 : canmsglib/CAN Unpack  CANdbFile=d:\Users\YJR\Desktop\DBC\SWAS.dbc  MsgList=(none)  MsgName=PPEI_Steering_Wheel_Angle  MsgIDType=Standard (11-bit identifier)  MsgIdentifier=330  MsgLength=8  SignalInfo={'StWhlAngAliveRollCnt','0','8','BE','unsigned','Standard','0','1','0','0','63';'StrWhAng','32','16','BE','unsigned','Standard','0','1.000000e-01','-7.793000e+02','-7.793000e+02','5.774200e+03';'StrWhAngV','16','8','BE','unsigned','Standard','0','1','0','0','1'}  IDPort=off  TimestampPort=off  ErrorPort=off  RemotePort=off  LengthPort=off  StatusPort=off  ApplyMinMax=off
      settings: SourceProductName=Simulink Real-Time  SourceProductBaseCode=XP  DataFormat=CANdb specified signals
  CANUnPackMessage4 : ec5744lib/RapidECU_U3/04CANCommunication/CANUnPackMessage  datalength=8  canmessagetype=Standard(11-bit ID)  sampletime=-1
      settings: SourceProductName=ECUCoder for MPC5744
  StrWhlAng : Outport  VectorParamsAs1DForOutWhenUnconnected=off
  StrWhlAngV : Outport  Port=2  VectorParamsAs1DForOutWhenUnconnected=off
  StrWhlAngAliveRollCnt : Outport  Port=3  VectorParamsAs1DForOutWhenUnconnected=off
  wires:
  Msg/1 -> CANUnPackMessage4/2
  ID/1 -> CANUnPackMessage4/1
  CANUnPackMessage4/1 -> CAN Unpack1/1
  CAN Unpack1/1 -> StrWhlAngAliveRollCnt/1
  CAN Unpack1/2 -> StrWhlAng/1
  CAN Unpack1/3 -> StrWhlAngV/1

== system INPUT_autosar/AMKMCU_Receive/FLAMKMCU/AMKMCU_state/MCU_state ==
  ID : Inport
  Msg : Inport  Port=2
  Enable : EnablePort
  Bus Creator : BusCreator  Inputs=12
  CAN Unpack : canmsglib/CAN Unpack  CANdbFile=d:\Users\YJR\Desktop\DBC\DRe20_dbc_v1.16\DRe20_dbc_v1.16_CAN2.dbc  MsgList=(none)  MsgName=MCFL_ActualValue1  MsgIDType=Standard (11-bit identifier)  MsgIdentifier=640  MsgLength=8  SignalInfo={'MCFL_ActualTorque','32','16','LE','signed','Standard','0','9.800000e-03','0','-Inf','Inf';'MCFL_ActualVelocity','48','16','LE','signed','Standard','0','1','0','-Inf','Inf';'MCFL_DCVoltage','16','16','LE','unsigned','Standard','0','1','0','-Inf','Inf';'MCFL_bDCOn','12','1','LE','unsigned','Standard','0','1','0','0','1';'MCFL_bDerating','15','1','LE','unsigned','Standard','0','1','0','0','1';'MCFL_bError','9','1','LE','unsigned','Standard','0','1','0','0','1';'MCFL_bInverterOn','14','1','LE','unsigned','Standard','0','1','0','0','1';'MCFL_bQuitDCOn','11','1','LE','unsigned','Standard','0','1','0','0','1';'MCFL_bQuitInverterOn','13','1','LE','unsigned','Standard','0','1','0','0','1';'MCFL_bReserve','0','8','LE','unsigned','Standard','0','1','0','0','255';'MCFL_bSystemReady','8','1','LE','unsigned','Standard','0','1','0','0','1';'MCFL_bWarn','10','1','LE','unsigned','Standard','0','1','0','0','1'}  IDPort=off  TimestampPort=off  ErrorPort=off  RemotePort=off  LengthPort=off  StatusPort=off  ApplyMinMax=off
      settings: SourceProductName=Simulink Real-Time  SourceProductBaseCode=XP  DataFormat=CANdb specified signals
  CANUnPackMessage4 : ec5744lib/RapidECU_U3/04CANCommunication/CANUnPackMessage  datalength=8  canmessagetype=Standard(11-bit ID)  sampletime=-1
      settings: SourceProductName=ECUCoder for MPC5744
  FLAMKMCUtoVCU1 : Outport  VectorParamsAs1DForOutWhenUnconnected=off
  wires:
  Msg/1 -> CANUnPackMessage4/2
  ID/1 -> CANUnPackMessage4/1
  CANUnPackMessage4/1 -> CAN Unpack/1
  CAN Unpack/1 -> Bus Creator/1  "MCFL_ActualTorque"
  CAN Unpack/2 -> Bus Creator/2  "MCFL_ActualVelocity"
  CAN Unpack/3 -> Bus Creator/3  "MCFL_DCVoltage"
  CAN Unpack/4 -> Bus Creator/4  "MCFL_bDCOn"
  CAN Unpack/5 -> Bus Creator/5  "MCFL_bDerating"
  CAN Unpack/6 -> Bus Creator/6  "MCFL_bError"
  CAN Unpack/7 -> Bus Creator/7  "MCFL_bInverterOn"
  CAN Unpack/8 -> Bus Creator/8  "MCFL_bQuitDCOn"
  CAN Unpack/9 -> Bus Creator/9  "MCFL_bQuitInverterOn"
  CAN Unpack/10 -> Bus Creator/10  "MCFL_bReserve"
  CAN Unpack/11 -> Bus Creator/11  "MCFL_bSystemReady"
  CAN Unpack/12 -> Bus Creator/12  "MCFL_bWarn"
  Bus Creator/1 -> FLAMKMCUtoVCU1/1  "FLAMKMCUtoVCU1"

== system INPUT_autosar/AMKMCU_Receive/FLAMKMCU/AMKMCU_state1/MCU_state ==
  ID : Inport
  Msg : Inport  Port=2
  Enable : EnablePort
  CAN Unpack : canmsglib/CAN Unpack  CANdbFile=d:\Users\YJR\Desktop\DBC\DRe20_dbc_v1.16\DRe20_dbc_v1.16_CAN2.dbc  MsgList=(none)  MsgName=MCFL_ActualValue2  MsgIDType=Standard (11-bit identifier)  MsgIdentifier=642  MsgLength=8  SignalInfo={'MCFL_DiagnosticNum','0','32','LE','unsigned','Standard','0','1','0','-Inf','Inf';'MCFL_ErrorInfo','32','32','LE','unsigned','Standard','0','1','0','-Inf','Inf'}  IDPort=off  TimestampPort=off  ErrorPort=off  RemotePort=off  LengthPort=off  StatusPort=off  ApplyMinMax=off
      settings: SourceProductName=Simulink Real-Time  SourceProductBaseCode=XP  DataFormat=CANdb specified signals
  CANUnPackMessage4 : ec5744lib/RapidECU_U3/04CANCommunication/CANUnPackMessage  datalength=8  canmessagetype=Standard(11-bit ID)  sampletime=-1
      settings: SourceProductName=ECUCoder for MPC5744
  MCFL_DiagnosticNum : Outport  VectorParamsAs1DForOutWhenUnconnected=off
  MCFL_ErrorInfo : Outport  Port=2  VectorParamsAs1DForOutWhenUnconnected=off
  wires:
  CANUnPackMessage4/1 -> CAN Unpack/1
  ID/1 -> CANUnPackMessage4/1
  Msg/1 -> CANUnPackMessage4/2
  CAN Unpack/1 -> MCFL_DiagnosticNum/1  "MCFL_DiagnosticNum"
  CAN Unpack/2 -> MCFL_ErrorInfo/1  "MCFL_ErrorInfo"

== system INPUT_autosar/AMKMCU_Receive/FLAMKMCU/AMKMCU_state2/MCU_state ==
  ID : Inport
  Msg : Inport  Port=2
  Enable : EnablePort
  CAN Unpack : canmsglib/CAN Unpack  CANdbFile=d:\Users\YJR\Desktop\DBC\DRe20_dbc_v1.16\DRe20_dbc_v1.16_CAN2.dbc  MsgList=(none)  MsgName=MCFL_ActualValue3  MsgIDType=Standard (11-bit identifier)  MsgIdentifier=644  MsgLength=6  SignalInfo={'MCFL_TempIGBT','32','16','LE','unsigned','Standard','0','1.000000e-01','0','-Inf','Inf';'MCFL_TempInverter','16','16','LE','unsigned','Standard','0','1.000000e-01','0','-Inf','Inf';'MCFL_TempMotor','0','16','LE','unsigned','Standard','0','1.000000e-01','0','-Inf','Inf'}  IDPort=off  TimestampPort=off  ErrorPort=off  RemotePort=off  LengthPort=off  StatusPort=off  ApplyMinMax=off
      settings: SourceProductName=Simulink Real-Time  SourceProductBaseCode=XP  DataFormat=CANdb specified signals
  CANUnPackMessage4 : ec5744lib/RapidECU_U3/04CANCommunication/CANUnPackMessage  datalength=8  canmessagetype=Standard(11-bit ID)  sampletime=-1
      settings: SourceProductName=ECUCoder for MPC5744
  MCFL_TempIGBT : Outport  VectorParamsAs1DForOutWhenUnconnected=off
  MCFL_TempInverter : Outport  Port=2  VectorParamsAs1DForOutWhenUnconnected=off
  MCFL_TempMotor : Outport  Port=3  VectorParamsAs1DForOutWhenUnconnected=off
  wires:
  Msg/1 -> CANUnPackMessage4/2
  ID/1 -> CANUnPackMessage4/1
  CANUnPackMessage4/1 -> CAN Unpack/1
  CAN Unpack/1 -> MCFL_TempIGBT/1  "MCFL_TempIGBT"
  CAN Unpack/2 -> MCFL_TempInverter/1  "MCFL_TempInverter"
  CAN Unpack/3 -> MCFL_TempMotor/1  "MCFL_TempMotor"

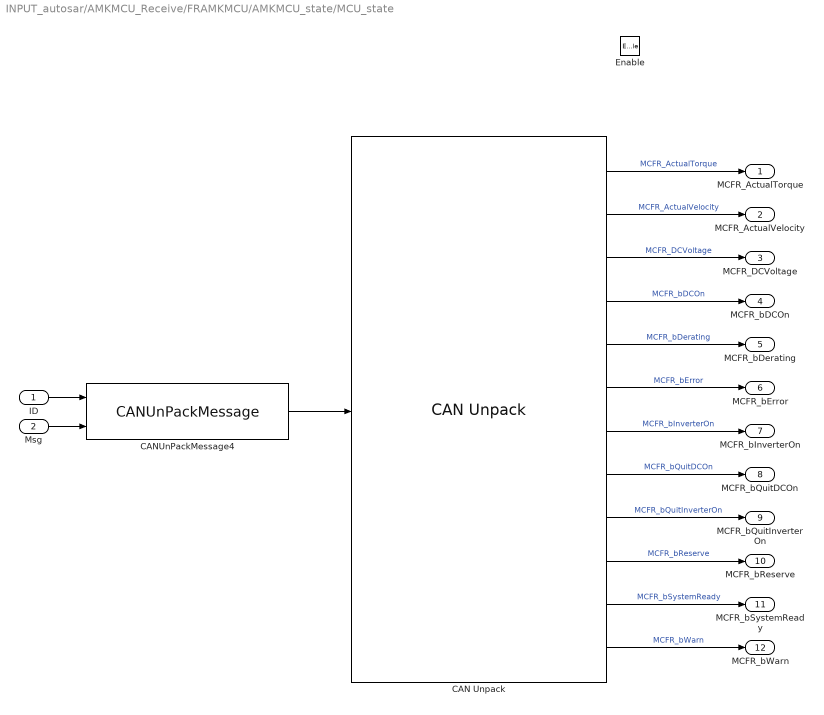
== system INPUT_autosar/AMKMCU_Receive/FRAMKMCU/AMKMCU_state/MCU_state ==
  ID : Inport
  Msg : Inport  Port=2
  Enable : EnablePort
  CAN Unpack : canmsglib/CAN Unpack  CANdbFile=d:\Users\YJR\Desktop\DBC\DRe20_dbc_v1.16\DRe20_dbc_v1.16_CAN2.dbc  MsgList=(none)  MsgName=MCFR_ActualValue1  MsgIDType=Standard (11-bit identifier)  MsgIdentifier=641  MsgLength=8  SignalInfo={'MCFR_ActualTorque','32','16','LE','signed','Standard','0','9.800000e-03','0','-Inf','Inf';'MCFR_ActualVelocity','48','16','LE','signed','Standard','0','1','0','-Inf','Inf';'MCFR_DCVoltage','16','16','LE','unsigned','Standard','0','1','0','-Inf','Inf';'MCFR_bDCOn','12','1','LE','unsigned','Standard','0','1','0','0','1';'MCFR_bDerating','15','1','LE','unsigned','Standard','0','1','0','0','1';'MCFR_bError','9','1','LE','unsigned','Standard','0','1','0','0','1';'MCFR_bInverterOn','14','1','LE','unsigned','Standard','0','1','0','0','1';'MCFR_bQuitDCOn','11','1','LE','unsigned','Standard','0','1','0','0','1';'MCFR_bQuitInverterOn','13','1','LE','unsigned','Standard','0','1','0','0','1';'MCFR_bReserve','0','8','LE','unsigned','Standard','0','1','0','0','255';'MCFR_bSystemReady','8','1','LE','unsigned','Standard','0','1','0','0','1';'MCFR_bWarn','10','1','LE','unsigned','Standard','0','1','0','0','1'}  IDPort=off  TimestampPort=off  ErrorPort=off  RemotePort=off  LengthPort=off  StatusPort=off  ApplyMinMax=off
      settings: SourceProductName=Simulink Real-Time  SourceProductBaseCode=XP  DataFormat=CANdb specified signals
  CANUnPackMessage4 : ec5744lib/RapidECU_U3/04CANCommunication/CANUnPackMessage  datalength=8  canmessagetype=Standard(11-bit ID)  sampletime=-1
      settings: SourceProductName=ECUCoder for MPC5744
  MCFR_ActualTorque : Outport  VectorParamsAs1DForOutWhenUnconnected=off
  MCFR_ActualVelocity : Outport  Port=2  VectorParamsAs1DForOutWhenUnconnected=off
  MCFR_DCVoltage : Outport  Port=3  VectorParamsAs1DForOutWhenUnconnected=off
  MCFR_bDCOn : Outport  Port=4  VectorParamsAs1DForOutWhenUnconnected=off
  MCFR_bDerating : Outport  Port=5  VectorParamsAs1DForOutWhenUnconnected=off
  MCFR_bError : Outport  Port=6  VectorParamsAs1DForOutWhenUnconnected=off
  MCFR_bInverterOn : Outport  Port=7  VectorParamsAs1DForOutWhenUnconnected=off
  MCFR_bQuitDCOn : Outport  Port=8  VectorParamsAs1DForOutWhenUnconnected=off
  MCFR_bQuitInverterOn : Outport  Port=9  VectorParamsAs1DForOutWhenUnconnected=off
  MCFR_bReserve : Outport  Port=10  VectorParamsAs1DForOutWhenUnconnected=off
  MCFR_bSystemReady : Outport  Port=11  VectorParamsAs1DForOutWhenUnconnected=off
  MCFR_bWarn : Outport  Port=12  VectorParamsAs1DForOutWhenUnconnected=off
  wires:
  CANUnPackMessage4/1 -> CAN Unpack/1
  ID/1 -> CANUnPackMessage4/1
  Msg/1 -> CANUnPackMessage4/2
  CAN Unpack/1 -> MCFR_ActualTorque/1  "MCFR_ActualTorque"
  CAN Unpack/2 -> MCFR_ActualVelocity/1  "MCFR_ActualVelocity"
  CAN Unpack/4 -> MCFR_bDCOn/1  "MCFR_bDCOn"
  CAN Unpack/3 -> MCFR_DCVoltage/1  "MCFR_DCVoltage"
  CAN Unpack/7 -> MCFR_bInverterOn/1  "MCFR_bInverterOn"
  CAN Unpack/5 -> MCFR_bDerating/1  "MCFR_bDerating"
  CAN Unpack/6 -> MCFR_bError/1  "MCFR_bError"
  CAN Unpack/8 -> MCFR_bQuitDCOn/1  "MCFR_bQuitDCOn"
  CAN Unpack/9 -> MCFR_bQuitInverterOn/1  "MCFR_bQuitInverterOn"
  CAN Unpack/10 -> MCFR_bReserve/1  "MCFR_bReserve"
  CAN Unpack/11 -> MCFR_bSystemReady/1  "MCFR_bSystemReady"
  CAN Unpack/12 -> MCFR_bWarn/1  "MCFR_bWarn"

== system INPUT_autosar/AMKMCU_Receive/FRAMKMCU/AMKMCU_state1/MCU_state ==
  ID : Inport
  Msg : Inport  Port=2
  Enable : EnablePort
  CAN Unpack : canmsglib/CAN Unpack  CANdbFile=d:\Users\YJR\Desktop\DBC\DRe20_dbc_v1.16\DRe20_dbc_v1.16_CAN2.dbc  MsgList=(none)  MsgName=MCFR_ActualValue2  MsgIDType=Standard (11-bit identifier)  MsgIdentifier=643  MsgLength=8  SignalInfo={'MCFR_DiagnosticNum','0','32','LE','unsigned','Standard','0','1','0','-Inf','Inf';'MCFR_ErrorInfo','32','32','LE','unsigned','Standard','0','1','0','-Inf','Inf'}  IDPort=off  TimestampPort=off  ErrorPort=off  RemotePort=off  LengthPort=off  StatusPort=off  ApplyMinMax=off
      settings: SourceProductName=Simulink Real-Time  SourceProductBaseCode=XP  DataFormat=CANdb specified signals
  CANUnPackMessage4 : ec5744lib/RapidECU_U3/04CANCommunication/CANUnPackMessage  datalength=8  canmessagetype=Standard(11-bit ID)  sampletime=-1
      settings: SourceProductName=ECUCoder for MPC5744
  MCFR_DiagnosticNum : Outport  VectorParamsAs1DForOutWhenUnconnected=off
  MCFR_ErrorInfo : Outport  Port=2  VectorParamsAs1DForOutWhenUnconnected=off
  wires:
  Msg/1 -> CANUnPackMessage4/2
  ID/1 -> CANUnPackMessage4/1
  CANUnPackMessage4/1 -> CAN Unpack/1
  CAN Unpack/1 -> MCFR_DiagnosticNum/1  "MCFR_DiagnosticNum"
  CAN Unpack/2 -> MCFR_ErrorInfo/1  "MCFR_ErrorInfo"
